simulink model "FLC"  (R2019a)
settings: Solver=ode45  StartTime=0.0  StopTime=10  RelTol=1e-3
libraries: fuzblock x1
settings Model: Creator=ansar  LastModifiedBy=ansar

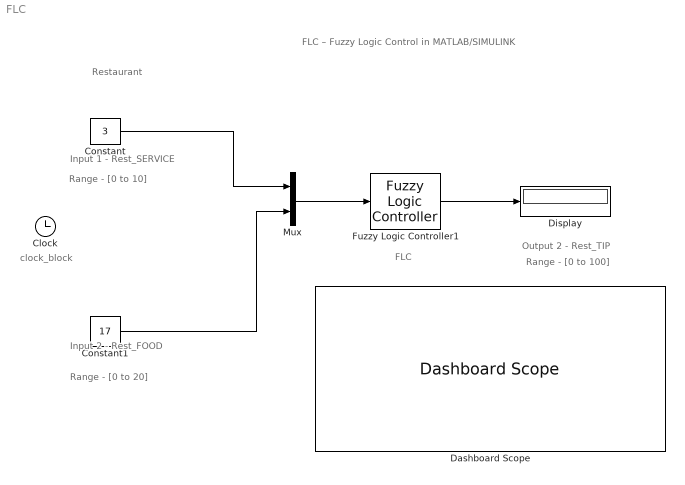
== system FLC ==
  note: clock_block
  note: Range - [0 to 20]
  note: Range - [0 to 10]
  note: FLC
  note: Range - [0 to 100]
  note: Output 2 - Rest_TIP
  note: Input 2 - Rest_FOOD
  note: Input 1 - Rest_SERVICE
  note: Restaurant
  note: FLC – Fuzzy Logic Control in MATLAB/SIMULINK
  Clock : Clock
  Constant : Constant  Value=3
  Constant1 : Constant  Value=17
  Dashboard Scope : DashboardScope
  Display : Display
  Fuzzy Logic Controller1 : fuzblock/Fuzzy Logic  Controller  FIS='Restaurant.fis'  OutputSampleNumber=101  DataType=double  FuzzifiedInputs=off  RuleFiringStrengths=off  RuleOutputs=off  AggregatedOutputs=off  SimulateUsing=Interpreted execution  OutOfRangeInputValueMessage=warning  NoRuleFiredMessage=warning  EmptyOutputFuzzySetMessage=warning
  Mux : Mux  Inputs=2
  wires:
  Fuzzy Logic Controller1/1 -> Display/1
  Mux/1 -> Fuzzy Logic Controller1/1
  Constant1/1 -> Mux/2
  Constant/1 -> Mux/1
